simulink model "zufall1"  (Simulink 4.00)
settings: Solver=ode45  StartTime=0.0  StopTime=5  RelTol=1e-3
settings Model: LastModifiedBy=Administrator  OutputOption=SpecifiedOutputTimes  OutputTimes=[0:0.1:5]  BlockReductionOpt=off

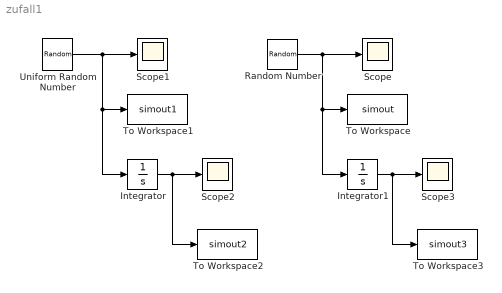
== system zufall1 ==
  Integrator : Integrator  ExternalReset=none  InitialConditionSource=internal  InitialCondition=0  LimitOutput=off  UpperSaturationLimit=inf  LowerSaturationLimit=-inf  ShowSaturationPort=off  ShowStatePort=off  AbsoluteTolerance=auto
  Integrator1 : Integrator  ExternalReset=none  InitialConditionSource=internal  InitialCondition=0  LimitOutput=off  UpperSaturationLimit=inf  LowerSaturationLimit=-inf  ShowSaturationPort=off  ShowStatePort=off  AbsoluteTolerance=auto
  Random Number : RandomNumber  Mean=[-1, 0, 1]  Variance=[0.3, 0.3, 0.3]  Seed=[138, 751, 97]  SampleTime=0
  Scope{,1..3} (4 alike) : Scope
      Scope settings: TimeRange=auto  YMin=-5  YMax=5  SaveToWorkspace=off  SaveName=ScopeData  LimitDataPoints=on  MaxDataPoints=5000
      Scope1 settings: TimeRange=auto  YMin=-5  YMax=5  SaveToWorkspace=off  LimitDataPoints=on  MaxDataPoints=5000
      Scope2 settings: TimeRange=auto  YMin=-5  YMax=5  SaveToWorkspace=off  SaveName=ScopeData2  LimitDataPoints=on  MaxDataPoints=5000
      Scope3 settings: TimeRange=auto  YMin=-5  YMax=5  SaveToWorkspace=off  SaveName=ScopeData3  LimitDataPoints=on  MaxDataPoints=5000
  To Workspace : ToWorkspace  VariableName=simout  SampleTime=-1  SaveFormat=Array
  To Workspace1 : ToWorkspace  VariableName=simout1  SampleTime=-1  SaveFormat=Array
  To Workspace2 : ToWorkspace  VariableName=simout2  SampleTime=-1  SaveFormat=Array
  To Workspace3 : ToWorkspace  VariableName=simout3  SampleTime=-1  SaveFormat=Array
  Uniform Random Number : UniformRandomNumber  Minimum=[-3,-1,1]  Maximum=[-1,1,3]  Seed=[7864, 0657, 1970]  SampleTime=0
  wires:
  Random Number/1 -> Scope/1, To Workspace/1, Integrator1/1
  Uniform Random Number/1 -> Scope1/1, To Workspace1/1, Integrator/1
  Integrator/1 -> Scope2/1, To Workspace2/1
  Integrator1/1 -> To Workspace3/1, Scope3/1
